simulink model "sgMdl_IO3xx_PWM_Loopback"  (R2024b)
settings: Solver=FixedStepAuto  StartTime=0.0  StopTime=inf  RelTol=1e-3  EnableMultiTasking=on
undefined symbols (not defined in the file): Pull, pull, Tpwm, Ts, up
libraries: speedgoatlib_fpga_pwm x5, speedgoatlib_fpga x1
Description:
  | PWM - Loopback
settings Model: ModifiedByFormat=Speedgoat  SimulationMode=external  ExtModeTrigDuration=100000  Creator=Speedgoat  LastModifiedBy=Speedgoat
settings SolverCC: ConcurrentTasks=on  AlgebraicLoopSolver=TrustRegion  PositivePriorityOrder=on  AutoInsertRateTranBlk=on  InsertRTBMode=Never (minimum delay)
settings DataIOCC: SaveFormat=StructureWithTime
settings OptimizationCC: BlockReduction=off  OptimizeBlockIOStorage=off  BufferReuse=off
settings DebuggingCC: UnderspecifiedInitializationDetection=Classic  MergeDetectMultiDrivingBlocksExec=none  TasksWithSamePriorityMsg=none
settings HardwareCC: ProdBitPerLong=64  ProdLongLongMode=on  ProdHWDeviceType=Intel->x86-64 (Linux 64)
settings ModelReferenceCC: EnableRefExpFcnMdlSchedulingChecks=on  PropagateSignalLabelsOutOfModel=off
settings RTWCC: Description=Speedgoat Real-Time Target Machine  SystemTargetFile=speedgoat.tlc  TLCOptions=-axpcCPUClockPoll=0  TemplateMakefile=slrealtime_default_tmf  Toolchain=Simulink Real-Time Toolchain  BuildConfiguration=Faster Runs  TargetLang=C++  GPUComputeCapability=3.5  DLArmComputeVersion=19.05
settings SimulinkRealTimeTargetCC: SubcomponentCodeInterfacePackaging=Reusable function  InstructionSetFMA=off  LogToMDFFile=off  SLRTFileLogMaxRuns=10  UseGCCFastMath=on
settings ConfigComp: CovBoundaryAbsTol=1.0e-5

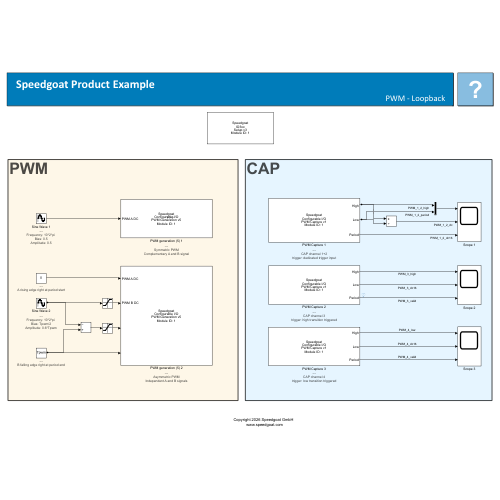
[thumbnail: Simulink's stored preview of the top-level diagram]
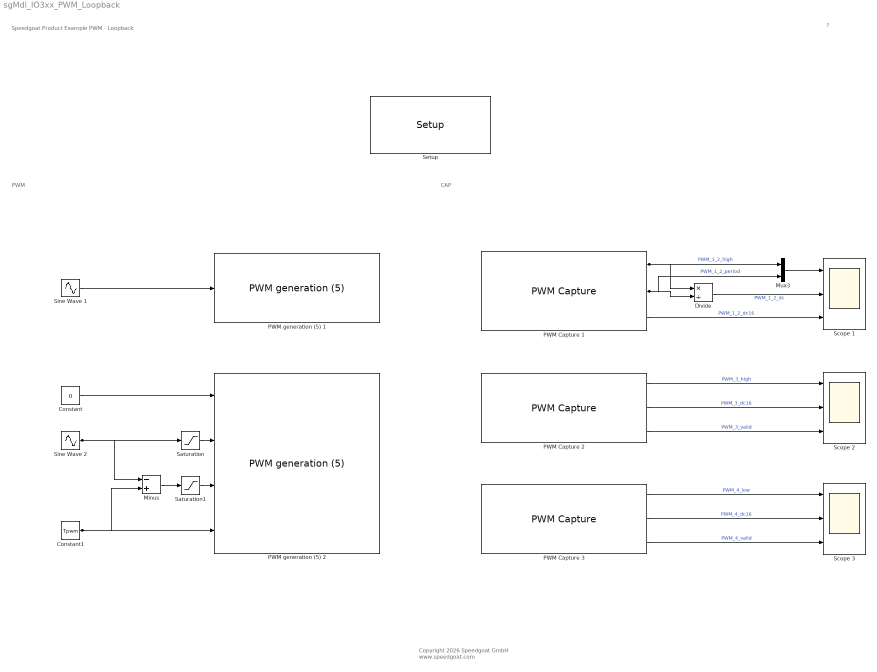
== system sgMdl_IO3xx_PWM_Loopback ==
  note: PWM
  note: CAP
  note: Speedgoat Product Example
      | PWM - Loopback
  note: ?
  note: Copyright 2026 Speedgoat GmbH
      |  www.speedgoat.com
  Constant : Constant  Value=0  SampleTime=Ts
      settings: AttributesFormatString=|
      | ---
      | A rising edge right at period start
  Constant1 : Constant  Value=Tpwm  SampleTime=Ts
      settings: AttributesFormatString=|
      | ---
      | B falling edge right at period end
  Divide : Product  Inputs=*/
  Minus : Sum  Inputs=-+
  Mux3 : Mux  Inputs=2
  PWM Capture 1 : speedgoatlib_fpga_pwm/PWM Capture  id=1  chan=[1,2]  ts=Ts  captureMode=Use dedicated trigger input  bit_width_cap=24  captureTimeout_si=0  captureTimeout_eff=0  debounce_si=100e-9  debounce_eff=106.7e-9  showHighDuration=on  showLowDuration=off  showPeriod=on  showDC16=on  showDC8=off  showTOn=off  showTOff=off  showValidData=off
      settings: SourceProductName=Simulink Real-Time: Speedgoat I/O Blockset
      settings: AttributesFormatString=|
      | ---
      | CAP channel 1+2
      | trigger: dedicated trigger input
  PWM Capture 2 : speedgoatlib_fpga_pwm/PWM Capture  id=1  chan=[3]  ts=Ts  captureMode=High transitions triggered  bit_width_cap=24  captureTimeout_si=1.1e-3  captureTimeout_eff=1.1e-3  debounce_si=10e-6  debounce_eff=10e-6  showHighDuration=on  showLowDuration=off  showPeriod=off  showDC16=on  showDC8=off  showTOn=off  showTOff=off  showValidData=on
      settings: SourceProductName=Simulink Real-Time: Speedgoat I/O Blockset
      settings: AttributesFormatString=|
      | ---
      | CAP channel 3
      | trigger: high transition triggered
  PWM Capture 3 : speedgoatlib_fpga_pwm/PWM Capture  id=1  chan=[4]  ts=Ts  captureMode=Low transitions triggered  bit_width_cap=24  captureTimeout_si=1.1e-3  captureTimeout_eff=1.1e-3  debounce_si=10e-6  debounce_eff=10e-6  showHighDuration=off  showLowDuration=on  showPeriod=off  showDC16=on  showDC8=off  showTOn=off  showTOff=off  showValidData=on
      settings: SourceProductName=Simulink Real-Time: Speedgoat I/O Blockset
      settings: AttributesFormatString=|
      | ---
      | CAP channel 4
      | trigger: low transition triggered
  PWM generation (5) 1 : speedgoatlib_fpga_pwm/PWM generation (5)  id=1  chan=[1]  board=Please select...  ts=Ts  pciSlot=-1  delay=0  symmetric=Symmetric - PWM generation is centered around half the period  b_is_complement_of_a=The complement of PWM A output  deadband=[0.0]  period=1e-3  frequency=1000  ticks=74999  a_on=[0]  a_off=[0]  pwm_a_dc=[0.0]  b_on=[0]  b_off=[0]  pwm_b_dc=[0]  c_on=[0.0]  c_off=[0.0]  protection=B is forced off when A is on.  enable_latch_half_period=off  pwm_update=At period starts  bit_width_pwm_gen=24  trigger_duration=[1e-6]  trigger_period_start=on  trigger_half_of_the_period=off  trigger_a_on=off  trigger_a_off=off  trigger_b_on=off  trigger_b_off=off  show_a_input=on  show_b_input=on  show_c_input=off  show_period_input=off  show_force_stop_input=off  idle_a=Low when PWM generation is halted  idle_b=Low when PWM generation is halted  idle_c=Low when PWM generation is halted  cancels_pwm_generation=on  invert_a=off  invert_b=off  invert_c=off
      settings: SourceProductName=Simulink Real-Time: Speedgoat I/O Blockset
      settings: AttributesFormatString=|
      | ---
      | Symmetric PWM
      | Complementary A and B signal
  PWM generation (5) 2 : speedgoatlib_fpga_pwm/PWM generation (5)  id=1  chan=[2]  board=Please select...  ts=Ts  pciSlot=-1  delay=0  symmetric=Asymmetric - On and Off are freely configurable  b_is_complement_of_a=Independent of PWM A output  deadband=[0.0]  period=1e-3  frequency=1000  ticks=74999  a_on=[0]  a_off=[0]  pwm_a_dc=[0.0]  b_on=[0]  b_off=[0]  pwm_b_dc=[0]  c_on=[0.0]  c_off=[0.0]  protection=Disabled: A and B can be high at the same moment  enable_latch_half_period=off  pwm_update=At period starts  bit_width_pwm_gen=24  trigger_duration=[1e-6]  trigger_period_start=off  trigger_half_of_the_period=off  trigger_a_on=off  trigger_a_off=off  trigger_b_on=off  trigger_b_off=off  show_a_input=on  show_b_input=on  show_c_input=off  show_period_input=off  show_force_stop_input=off  idle_a=Low when PWM generation is halted  idle_b=Low when PWM generation is halted  idle_c=Low when PWM generation is halted  cancels_pwm_generation=on  invert_a=off  invert_b=off  invert_c=off
      settings: SourceProductName=Simulink Real-Time: Speedgoat I/O Blockset
      settings: AttributesFormatString=|
      | ---
      | Asymmetric PWM
      | Independent A and B signals
  Saturation : Saturate  UpperLimit=Tpwm  LowerLimit=0
  Saturation1 : Saturate  UpperLimit=Tpwm  LowerLimit=0
  Scope 1 : Scope  NumInputPorts=3
  Scope 2 : Scope  NumInputPorts=3
  Scope 3 : Scope  NumInputPorts=3
  Setup : speedgoatlib_fpga/Setup/Setup  board=Please select...  id=1  pciSlot=-1  device_id=1  bitstreamFilePath=[]  bitstreamFile=<Manual entry>  fpgaFreq=75 MHz  enableDma=off  rearEnb_1=off  rearIO_1=None  rearEnb_2=off  rearIO_2=None  ProgSpiFlash=off  ProgBPIFlash=off  useFpgaDmaController=off  dmaTrigDropdown=Model Step  dmaTrigSelect=0  dmaStopOnOverload=on  dmaModeSequential=on  dmaModeParallel=off  PullRPort15=pull-up 3.3V  PullRPort31=pull-up 3.3V  PullRPort47=pull-up 3.3V  PullRPort63=pull-up 3.3V  diffLineTermination_1=on  diffLineTermination_2=on  diffLineTermination_3=on  diffLineTermination_4=on  diffLineTermination_5=on  diffLineTermination_6=on  diffLineTermination_7=on  diffLineTermination_8=on  diffLineTermination_9=on  diffLineTermination_10=on  diffLineTermination_11=on  diffLineTermination_12=on  diffLineTermination_13=on  diffLineTermination_14=on  diffLineTermination_15=on  diffLineTermination_16=on  diffLineTermination_17=on  diffLineTermination_18=on  diffLineTermination_19=on  diffLineTermination_20=on  diffLineTermination_21=on  diffLineTermination_22=on  diffLineTermination_23=on  diffLineTermination_24=on  diffLineTermination_25=on  diffLineTermination_26=on  diffLineTermination_27=on  diffLineTermination_28=on  diffLineTermination_29=on  diffLineTermination_30=on  diffLineTermination_31=on  diffLineTermination_32=on  ioVoltageDropDown1=3.3V  pullResistorDropDown1_1=Pull-up  pullResistorDropDown1_2=Pull-up  pullResistorDropDown1_3=Pull-up  pullResistorDropDown1_4=Pull-up  pullResistorDropDown1_5=Pull-up  pullResistorDropDown1_6=Pull-up  pullResistorDropDown1_7=Pull-up  pullResistorDropDown1_8=Pull-up  ttlIsImplementedCheckBox1=off  pullResistorDropDown2=Pull-up  ioVoltageDropDown2=3.3V  ttlIsImplementedCheckBox2=off  pullResistorDropDown3=Pull-up  ioVoltageDropDown3=3.3V  ttlIsImplementedCheckBox3=off  pullResistorDropDown4=Pull-up  ioVoltageDropDown4=3.3V  ttlIsImplementedCheckBox4=off  pullResistorDropDown5=Pull-up  ioVoltageDropDown5=3.3V  ttlIsImplementedCheckBox5=off  pullResistorDropDown6=Pull-up  ioVoltageDropDown6=3.3V  ttlIsImplementedCheckBox6=off  pullResistorDropDown7=Pull-up  ioVoltageDropDown7=3.3V  ttlIsImplementedCheckBox7=off  pullResistorDropDown8=Pull-up  ioVoltageDropDown8=3.3V  ttlIsImplementedCheckBox8=off  terminationCheckBox1=off  terminationCheckBox2=off  terminationCheckBox3=off  terminationCheckBox4=off  diffIsImplementedCheckBox1=off  terminationCheckBox5=off  terminationCheckBox6=off  terminationCheckBox7=off  terminationCheckBox8=off  diffIsImplementedCheckBox2=off  terminationCheckBox9=off  terminationCheckBox10=off  terminationCheckBox11=off  terminationCheckBox12=off  diffIsImplementedCheckBox3=off  terminationCheckBox13=off  terminationCheckBox14=off  terminationCheckBox15=off  terminationCheckBox16=off  diffIsImplementedCheckBox4=off  terminationCheckBox17=off  terminationCheckBox18=off  terminationCheckBox19=off  terminationCheckBox20=off  diffIsImplementedCheckBox5=off  terminationCheckBox21=off  terminationCheckBox22=off  terminationCheckBox23=off  terminationCheckBox24=off  diffIsImplementedCheckBox6=off  terminationCheckBox25=off  terminationCheckBox26=off  terminationCheckBox27=off  terminationCheckBox28=off  diffIsImplementedCheckBox7=off  terminationCheckBox29=off  terminationCheckBox30=off  terminationCheckBox31=off  terminationCheckBox32=off  diffIsImplementedCheckBox8=off  PullRPort0_1=pull-up  VioPort0_1=3.3V  PullRPort1_1=pull-up  VioPort1_1=3.3V  PullRPort2_1=pull-up  VioPort2_1=3.3V  PullRPort3_1=pull-up  VioPort3_1=3.3V  PullRPort4_1=pull-up  VioPort4_1=3.3V  PullRPort5_1=pull-up  VioPort5_1=3.3V  PullRPort6_1=pull-up  VioPort6_1=3.3V  diffLineTermination_rear1_1=on  diffLineTermination_rear1_2=on  diffLineTermination_rear1_3=on  diffLineTermination_rear1_4=on  diffLineTermination_rear1_5=on  diffLineTermination_rear1_6=on  diffLineTermination_rear1_7=on  diffLineTermination_rear1_8=on  PullRPort0_2=pull-up  VioPort0_2=3.3V  PullRPort1_2=pull-up  VioPort1_2=3.3V  PullRPort2_2=pull-up  VioPort2_2=3.3V  PullRPort3_2=pull-up  VioPort3_2=3.3V  PullRPort4_2=pull-up  VioPort4_2=3.3V  PullRPort5_2=pull-up  VioPort5_2=3.3V  PullRPort6_2=pull-up  VioPort6_2=3.3V  diffLineTermination_rear2_1=on  diffLineTermination_rear2_2=on  diffLineTermination_rear2_3=on  diffLineTermination_rear2_4=on  diffLineTermination_rear2_5=on  diffLineTermination_rear2_6=on  diffLineTermination_rear2_7=on  diffLineTermination_rear2_8=on
      settings: SourceProductName=Simulink Real-Time: Speedgoat Library
  Sine Wave 1 : Sin  Amplitude=0.5  Bias=0.5  Frequency=10*2*pi  SampleTime=Ts
      settings: AttributesFormatString=|
      | ---
      | Frequency: %<Frequency>
      | Bias: %<Bias>
      | Amplitude: %<Amplitude>
  Sine Wave 2 : Sin  Amplitude=0.6*Tpwm  Bias=Tpwm/2  Frequency=10*2*pi  SampleTime=Ts
      settings: AttributesFormatString=|
      | ---
      | Frequency: %<Frequency>
      | Bias: %<Bias>
      | Amplitude: %<Amplitude>
  wires:
  Constant/1 -> PWM generation (5) 2/1
  Constant1/1 -> PWM generation (5) 2/4, Minus/2
  Sine Wave 2/1 -> Minus/1, Saturation/1
  Minus/1 -> Saturation1/1
  Sine Wave 1/1 -> PWM generation (5) 1/1
  PWM Capture 3/1 -> Scope 3/1  "PWM_4_low"
  PWM Capture 3/2 -> Scope 3/2  "PWM_4_dc16"
  PWM Capture 1/2 -> Divide/2, Mux3/2  "PWM_1_2_period"
  PWM Capture 1/1 -> Divide/1, Mux3/1  "PWM_1_2_high"
  Divide/1 -> Scope 1/2  "PWM_1_2_dc"
  PWM Capture 1/3 -> Scope 1/3  "PWM_1_2_dc16"
  Mux3/1 -> Scope 1/1
  Saturation/1 -> PWM generation (5) 2/2
  Saturation1/1 -> PWM generation (5) 2/3
  PWM Capture 3/3 -> Scope 3/3  "PWM_4_valid"
  PWM Capture 2/1 -> Scope 2/1  "PWM_3_high"
  PWM Capture 2/2 -> Scope 2/2  "PWM_3_dc16"
  PWM Capture 2/3 -> Scope 2/3  "PWM_3_valid"
